simulink model "PresaDepredador_lineal"  (R2021b)
settings: Solver=ode45  StartTime=0.0  StopTime=Time  RelTol=1e-7
undefined symbols (not defined in the file): A, alpha, Amplitude, B, beta, C, D, D0, delta, Frequency, gamma, N_eq, P0, ul
settings Model: Creator=curie  LastModifiedBy=alex
settings SolverCC: AlgebraicLoopSolver=TrustRegion
settings DataIOCC: ReturnWorkspaceOutputs=off
settings DebuggingCC: SFMachineParentedDataDiag=warning

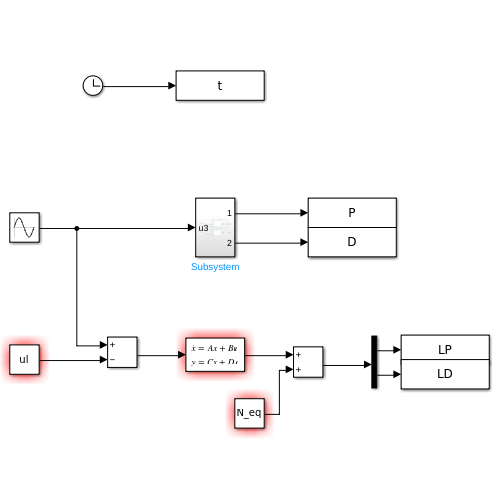
[thumbnail: Simulink's stored preview of the top-level diagram]
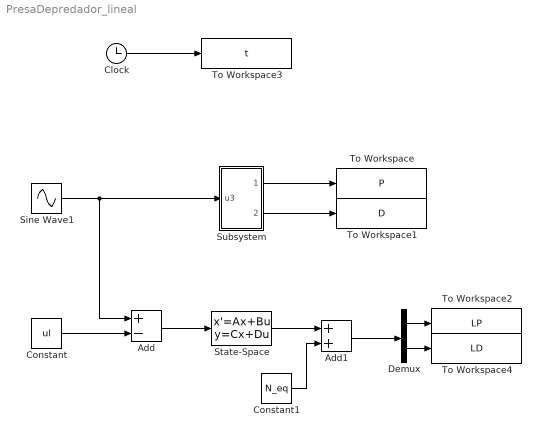
== system PresaDepredador_lineal ==
  Add : Sum  Inputs=+-
  Add1 : Sum
  Clock : Clock
  Constant : Constant  Value=ul
  Constant1 : Constant  Value=N_eq
  Demux : Demux  Outputs=2
  Sine Wave1 : Sin  Amplitude=Amplitude  Bias=u  Frequency=Frequency  SampleTime=0
  State-Space : StateSpace  A=A  B=B  C=C  D=D  InitialCondition=[0,0]
  Subsystem : Subsystem
  To Workspace : ToWorkspace  VariableName=P  SampleTime=-1
  To Workspace1 : ToWorkspace  VariableName=D  SampleTime=-1
  To Workspace2 : ToWorkspace  VariableName=LP  SampleTime=-1
  To Workspace3 : ToWorkspace  VariableName=t  SampleTime=-1
  To Workspace4 : ToWorkspace  VariableName=LD  SampleTime=-1
  wires:
  Subsystem/1(Out1) -> To Workspace/1
  Subsystem/2(Out2) -> To Workspace1/1
  Sine Wave1/1 -> Subsystem/1(u3), Add/1
  Clock/1 -> To Workspace3/1
  Add/1 -> State-Space/1
  Constant/1 -> Add/2
  State-Space/1 -> Add1/1
  Constant1/1 -> Add1/2
  Add1/1 -> Demux/1
  Demux/2 -> To Workspace4/1
  Demux/1 -> To Workspace2/1

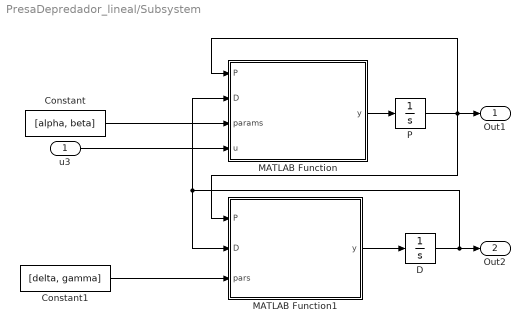
== system PresaDepredador_lineal/Subsystem ==
  u3 : Inport
  Constant : Constant  Value=[alpha, beta]
  Constant1 : Constant  Value=[delta, gamma]
  D : Integrator  InitialCondition=D0
  MATLAB Function : MATLAB Function  TreatAsAtomicUnit=on
  MATLAB Function1 : MATLAB Function  TreatAsAtomicUnit=on
  P : Integrator  InitialCondition=P0
  Out1 : Outport
  Out2 : Outport  Port=2
  wires:
  MATLAB Function/1(y) -> P/1
  D/1 -> MATLAB Function/2(D), MATLAB Function1/2(D), Out2/1
  MATLAB Function1/1(y) -> D/1
  Constant1/1 -> MATLAB Function1/3(pars)
  P/1 -> MATLAB Function/1(P), Out1/1, MATLAB Function1/1(P)
  Constant/1 -> MATLAB Function/3(params)
  u3/1 -> MATLAB Function/4(u)

== matlab function PresaDepredador_lineal/Subsystem/MATLAB Function1 ==
  data: P input; y output; D input; pars input
function y = fcn(P,D,pars)

delta = pars(1);
gamma = pars(2);

y = delta*P*D-gamma*D;

== matlab function PresaDepredador_lineal/Subsystem/MATLAB Function ==
  data: P input; D input; params input; u input; y output
function y = fcn(P,D,params,u)

    alpha=params(1);
    beta = params(2);

y = alpha*P-beta*D*P+u;
